simulink model "Tutorial25"  (R2020a)
settings: Solver=FixedStepDiscrete  StartTime=0.0  StopTime=20  FixedStep=1  RelTol=1e-3
libraries: simulink x1
settings Model: Creator=ashok  LastModifiedBy=ashok

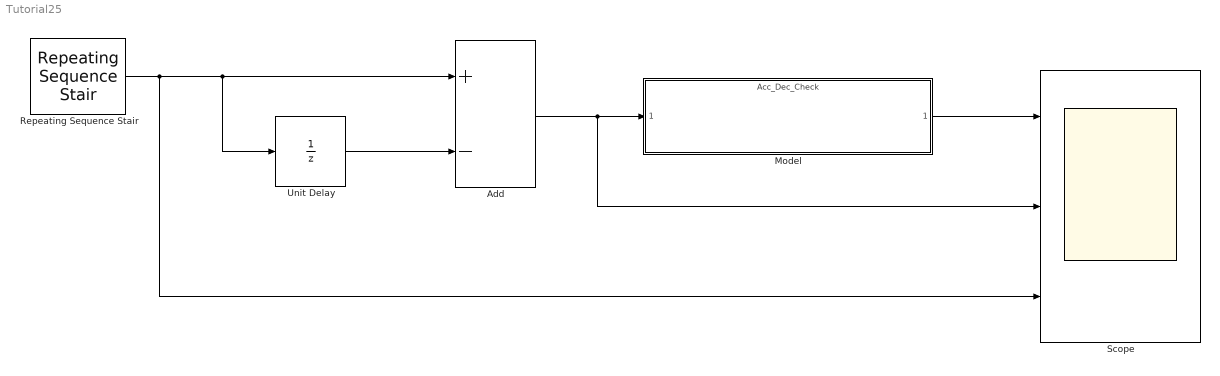
== system Tutorial25 ==
  Add : Sum  Inputs=+-
  Model : ModelReference  ModelNameDialog=Acc_Dec_Check  SimulationMode=Normal  ModelReferenceVersion=1.4
  Repeating Sequence Stair : simulink/Sources/Repeating Sequence Stair  OutValues=[3 1 4 2 1 -3 1 7 2 -1 -8 -2 -4].'  tsamp=-1  OutMin=[]  OutMax=[]  OutDataTypeStr=double  OutputDataTypeScalingMode=double  OutDataType=fixdt(0,8)  ConRadixGroup=Best Precision: Vector-wise  OutScaling=2^-12
  Scope : Scope  NumInputPorts=3
  Unit Delay : UnitDelay  SampleTime=-1  HasFrameUpgradeWarning=on
  wires:
  Repeating Sequence Stair/1 -> Scope/3, Unit Delay/1, Add/1
  Unit Delay/1 -> Add/2
  Add/1 -> Scope/2, Model/1
  Model/1 -> Scope/1
